simulink model "SF015A_WhlImbRejctn"  (R2013b)
settings: Solver=FixedStepDiscrete  SolverMode=SingleTasking  StartTime=0.0  StopTime=1  FixedStep=0.002  RelTol=1e-3
values from neighbouring files (symbols this model uses):
  ACTIVBANDMAX_ULS_U32 = DataDict.Constant    [SF015A_WhlImbRejctn_DataDict.m]
  ADAPVFILMAX_ULS_F32 = DataDict.Constant    [SF015A_WhlImbRejctn_DataDict.m]
  ARCHGLBPRM_180OVERPI_ULS_F32 = DataDict.Constant    [SF015A_WhlImbRejctn_DataDict.m]
  ARCHGLBPRM_2MILLISEC_SEC_F32 = DataDict.Constant    [SF015A_WhlImbRejctn_DataDict.m]
  ARCHGLBPRM_2PI_ULS_F32 = DataDict.Constant    [SF015A_WhlImbRejctn_DataDict.m]
  ARCHGLBPRM_FLOATZEROTHD_ULS_F32 = DataDict.Constant    [SF015A_WhlImbRejctn_DataDict.m]
  ARCHGLBPRM_PI_ULS_F32 = DataDict.Constant    [SF015A_WhlImbRejctn_DataDict.m]
  ARCHGLBPRM_PIOVER180_ULS_F32 = DataDict.Constant    [SF015A_WhlImbRejctn_DataDict.m]
  ARCHGLBPRM_PIOVER2_ULS_F32 = DataDict.Constant    [SF015A_WhlImbRejctn_DataDict.m]
  CALMINSPERCOUNT_ULS_F32 = DataDict.Constant    [SF015A_WhlImbRejctn_DataDict.m]
  DURATIONDISABLE_CNT_U16 = DataDict.Constant    [SF015A_WhlImbRejctn_DataDict.m]
  FILTWHLSPDMAX_MOTRADPERSEC_F32 = DataDict.Constant    [SF015A_WhlImbRejctn_DataDict.m]
  MICROSECTOMILLISEC_ULS_F32 = DataDict.Constant    [SF015A_WhlImbRejctn_DataDict.m]
  MINSTOMILLISEC_ULS_F32 = DataDict.Constant    [SF015A_WhlImbRejctn_DataDict.m]
  NINETY_ULS_F32 = DataDict.Constant    [SF015A_WhlImbRejctn_DataDict.m]
  NODEBSTEP_CNT_U16 = DataDict.Constant    [SF015A_WhlImbRejctn_DataDict.m]
  NROFDLY_CNT_U08 = DataDict.Constant    [SF015A_WhlImbRejctn_DataDict.m]
  ONEHALF_ULS_F32 = DataDict.Constant    [SF015A_WhlImbRejctn_DataDict.m]
  ONEHUNDRED_ULS_F32 = DataDict.Constant    [SF015A_WhlImbRejctn_DataDict.m]
  ONEOVRTHREE_ULS_F32 = DataDict.Constant    [SF015A_WhlImbRejctn_DataDict.m]
  ONEOVRTWENTY_ULS_F32 = DataDict.Constant    [SF015A_WhlImbRejctn_DataDict.m]
  ONETHOUSAND_ULS_F32 = DataDict.Constant    [SF015A_WhlImbRejctn_DataDict.m]
  PEAKMAX_ULS_F32 = DataDict.Constant    [SF015A_WhlImbRejctn_DataDict.m]
  PEAKMIN_ULS_F32 = DataDict.Constant    [SF015A_WhlImbRejctn_DataDict.m]
  PHAADJMAX_ULS_F32 = DataDict.Constant    [SF015A_WhlImbRejctn_DataDict.m]
  PITIMESSAMPLETIME_ULS_F32 = DataDict.Constant    [SF015A_WhlImbRejctn_DataDict.m]
  STOREDMINSPERCOUNT_ULS_F32 = DataDict.Constant    [SF015A_WhlImbRejctn_DataDict.m]
  TWO_ULS_F32 = DataDict.Constant    [SF015A_WhlImbRejctn_DataDict.m]
  TWOOVRTHREE_ULS_F32 = DataDict.Constant    [SF015A_WhlImbRejctn_DataDict.m]
  WhlImbRejctnAdpvFac = DataDict.Calibration    [SF015A_WhlImbRejctn_DataDict.m]
  WhlImbRejctnAutScaEna = DataDict.Calibration    [SF015A_WhlImbRejctn_DataDict.m]
  WhlImbRejctnAutScaTar = DataDict.Calibration    [SF015A_WhlImbRejctn_DataDict.m]
  WhlImbRejctnCurrMgnSlewPerLoop = DataDict.Calibration    [SF015A_WhlImbRejctn_DataDict.m]
  WhlImbRejctnDcTrendFltRcvryDly = DataDict.Calibration    [SF015A_WhlImbRejctn_DataDict.m]
  WhlImbRejctnDcTrendFltRcvryNegStep = DataDict.Calibration    [SF015A_WhlImbRejctn_DataDict.m]
  WhlImbRejctnDcTrendFltRcvryPosStep = DataDict.Calibration    [SF015A_WhlImbRejctn_DataDict.m]
  WhlImbRejctnDcTrendFltRcvryThd = DataDict.Calibration    [SF015A_WhlImbRejctn_DataDict.m]
  WhlImbRejctnDcTrendTh2Tq = DataDict.Calibration    [SF015A_WhlImbRejctn_DataDict.m]
  WhlImbRejctnDcTrendThTq = DataDict.Calibration    [SF015A_WhlImbRejctn_DataDict.m]
  WhlImbRejctnDcTrendTi2Sec = DataDict.Calibration    [SF015A_WhlImbRejctn_DataDict.m]
  WhlImbRejctnDcTrendTiSec = DataDict.Calibration    [SF015A_WhlImbRejctn_DataDict.m]
  WhlImbRejctnEnaSlewPerLoop = DataDict.Calibration    [SF015A_WhlImbRejctn_DataDict.m]
  WhlImbRejctnFctEna = DataDict.Calibration    [SF015A_WhlImbRejctn_DataDict.m]
  WhlImbRejctnFrqDiagcAmpThd = DataDict.Calibration    [SF015A_WhlImbRejctn_DataDict.m]
  WhlImbRejctnFrqDiagcEna = DataDict.Calibration    [SF015A_WhlImbRejctn_DataDict.m]
  WhlImbRejctnFrqDiagcFltRcvryDly = DataDict.Calibration    [SF015A_WhlImbRejctn_DataDict.m]
  WhlImbRejctnFrqDiagcFltRcvryNegStep = DataDict.Calibration    [SF015A_WhlImbRejctn_DataDict.m]
  WhlImbRejctnFrqDiagcFltRcvryPosStep = DataDict.Calibration    [SF015A_WhlImbRejctn_DataDict.m]
  WhlImbRejctnFrqDiagcFltRcvryThd = DataDict.Calibration    [SF015A_WhlImbRejctn_DataDict.m]
  WhlImbRejctnFrqDiagcThd = DataDict.Calibration    [SF015A_WhlImbRejctn_DataDict.m]
  WhlImbRejctnFrqDiagcTout = DataDict.Calibration    [SF015A_WhlImbRejctn_DataDict.m]
  WhlImbRejctnFrqDiagcUgrPoleMgn = DataDict.Calibration    [SF015A_WhlImbRejctn_DataDict.m]
  WhlImbRejctnFrqScaTblX = DataDict.Calibration    [SF015A_WhlImbRejctn_DataDict.m]
  WhlImbRejctnMaxDurn = DataDict.Calibration    [SF015A_WhlImbRejctn_DataDict.m]
  WhlImbRejctnMaxMgn = DataDict.Calibration    [SF015A_WhlImbRejctn_DataDict.m]
  WhlImbRejctnMaxMgnFltNegStep = DataDict.Calibration    [SF015A_WhlImbRejctn_DataDict.m]
  WhlImbRejctnMaxMgnFltPosStep = DataDict.Calibration    [SF015A_WhlImbRejctn_DataDict.m]
  WhlImbRejctnMaxMgnFltRcvryDly = DataDict.Calibration    [SF015A_WhlImbRejctn_DataDict.m]
  WhlImbRejctnMaxMgnFltRcvryNegStep = DataDict.Calibration    [SF015A_WhlImbRejctn_DataDict.m]
  WhlImbRejctnMaxMgnFltRcvryPosStep = DataDict.Calibration    [SF015A_WhlImbRejctn_DataDict.m]
  WhlImbRejctnMaxMgnFltRcvryThd = DataDict.Calibration    [SF015A_WhlImbRejctn_DataDict.m]
  WhlImbRejctnMaxMgnFltThd = DataDict.Calibration    [SF015A_WhlImbRejctn_DataDict.m]
  WhlImbRejctnMgnEstimnDeltaSca = DataDict.Calibration    [SF015A_WhlImbRejctn_DataDict.m]
  WhlImbRejctnMgnEstimnDiThd = DataDict.Calibration    [SF015A_WhlImbRejctn_DataDict.m]
  WhlImbRejctnMgnEstimnEnaThd = DataDict.Calibration    [SF015A_WhlImbRejctn_DataDict.m]
  WhlImbRejctnMgnEstimnFrq = DataDict.Calibration    [SF015A_WhlImbRejctn_DataDict.m]
  WhlImbRejctnMgnEstimnFrqDelta = DataDict.Calibration    [SF015A_WhlImbRejctn_DataDict.m]
  WhlImbRejctnMgnEstimnLeak = DataDict.Calibration    [SF015A_WhlImbRejctn_DataDict.m]
  WhlImbRejctnRampDwnTi = DataDict.Calibration    [SF015A_WhlImbRejctn_DataDict.m]
  WhlImbRejctnScaCncl = DataDict.Calibration    [SF015A_WhlImbRejctn_DataDict.m]
  WhlImbRejctnUgrPoleMgn = DataDict.Calibration    [SF015A_WhlImbRejctn_DataDict.m]
  WhlImbRejctnVehSpdEna = DataDict.Calibration    [SF015A_WhlImbRejctn_DataDict.m]
  WhlImbRejctnWhlSpdCorrlnFltRcvryDly = DataDict.Calibration    [SF015A_WhlImbRejctn_DataDict.m]
  WhlImbRejctnWhlSpdCorrlnFltRcvryNegStep = DataDict.Calibration    [SF015A_WhlImbRejctn_DataDict.m]
  WhlImbRejctnWhlSpdCorrlnFltRcvryPosStep = DataDict.Calibration    [SF015A_WhlImbRejctn_DataDict.m]
  WhlImbRejctnWhlSpdCorrlnFltRcvryThd = DataDict.Calibration    [SF015A_WhlImbRejctn_DataDict.m]
  WhlImbRejctnWhlSpdCorrlnThd = DataDict.Calibration    [SF015A_WhlImbRejctn_DataDict.m]
  WhlImbRejctnWhlSpdCorrlnTi = DataDict.Calibration    [SF015A_WhlImbRejctn_DataDict.m]
  WIRCMDMAX_MOTNWTMTR_F32 = DataDict.Constant    [SF015A_WhlImbRejctn_DataDict.m]
  ZERO_ULS_F32 = DataDict.Constant    [SF015A_WhlImbRejctn_DataDict.m]
undefined symbols (not defined in the file or in its folder): Cntr, NtcNr1, NvmGetErrSts1, SigQlfr1, Sts, SysSt1
libraries: simulink x32, FixdToFloat x32, Fil x20, NxtrLim x15, NxtrNvM x12, NxtrAbslt x8, NxtrMath x7, NxtrMax x6, NxtrMin x4, FloatToFixd x2, LnrIntrpn x2, NxtrSign x1
(part 1 of 12)
settings Model: Creator=VZBTJX  LastModifiedBy=VZBTJX
settings SolverCC: AutoInsertRateTranBlk=on  InsertRTBMode=Always
settings DataIOCC: LimitDataPoints=off  SaveFormat=Structure  ReturnWorkspaceOutputs=on
settings OptimizationCC: BlockReduction=off  InlineParams=on  ZeroExternalMemoryAtStartup=off  ZeroInternalMemoryAtStartup=off  OptimizeModelRefInitCode=on  LifeSpan=1
settings DebuggingCC: SignalInfNanChecking=error  SignalRangeChecking=warning  UnderspecifiedInitializationDetection=Simplified  SolverPrmCheckMsg=error  InheritedTsInSrcMsg=error  DiscreteInheritContinuousMsg=error  SingleTaskRateTransMsg=error  TasksWithSamePriorityMsg=error  SigSpecEnsureSampleTimeMsg=error  CheckMatrixSingularityMsg=error  ParameterUnderflowMsg=error  ParameterPrecisionLossMsg=error  ParameterTunabilityLossMsg=error  FixptConstUnderflowMsg=warning  FixptConstOverflowMsg=warning  VectorMatrixConversionMsg=error  SignalLabelMismatchMsg=error  UnconnectedInputMsg=error  UnconnectedOutputMsg=error  UnconnectedLineMsg=error  SFcnCompatibilityMsg=error  UniqueDataStoreMsg=warning  BusObjectLabelMismatch=error  RootOutportRequireBusObject=error  AssertControl=DisableAll  ModelReferenceIOMsg=error  ModelReferenceVersionMismatchMessage=warning  ModelReferenceIOMismatchMessage=error  ModelReferenceCSMismatchMessage=warning  ModelReferenceDataLoggingMessage=error  StateNameClashWarn=warning  StrictBusMsg=ErrorOnBusTreatedAsVector  NonBusSignalsTreatedAsBus=error  SFUnexpectedBacktrackingDiag=error  SFInvalidInputDataAccessInChartInitDiag=error  SFNoUnconditionalDefaultTransitionDiag=error  SFTransitionOutsideNaturalParentDiag=error  SFUnconditionalTransitionShadowingDiag=error  SFUndirectedBroadcastEventsDiag=error
settings ModelReferenceCC: ModelReferenceNumInstancesAllowed=Single
settings RTWCC: SystemTargetFile=autosar.tlc  GenCodeOnly=on  TemplateMakefile=ert_default_tmf  Description=AUTOSAR  GenerateReport=on  ProcessScript=autosar_make_rtw_hook  LaunchReport=on
settings CodeAppCC: GenerateComments=off  IgnoreCustomStorageClasses=off  CustomSymbolStrType=$N$R$M  CustomSymbolStrBlkIO=$N$M  SimulinkBlockComments=off
settings STFCustomTargetCC: ParMdlRefBuildCompliant=on  CompOptLevelCompliant=on  IncludeMdlTerminateFcn=off  CombineOutputUpdateFcns=on  SuppressErrorStatus=on  ERTFirstTimeCompliant=on  ERTCustomFileBanners=on  SupportNonFinite=off  SupportComplex=off  SupportContinuousTime=off  SupportNonInlinedSFcns=off  MATLABClassNameForMDSCustomization=Simulink.SoftwareTarget.ERTCustomization  AutosarCompliant=on  GRTInterface=off  SystemTargetFile=autosar.tlc
settings ERTTargetCC: CodeReplacementLibrary=ANSI_C  ConcurrentExecutionCompliant=off  IncludeMdlTerminateFcn=off  SuppressErrorStatus=on  SupportNonFinite=off  SupportComplex=off  ModelStepFunctionPrototypeControlCompliant=off  CPPClassGenCompliant=off  AutosarCompliant=on  InlinedParameterPlacement=NonHierarchical  ERTCustomFileTemplate=example_file_process.tlc  EnableUserReplacementTypes=on

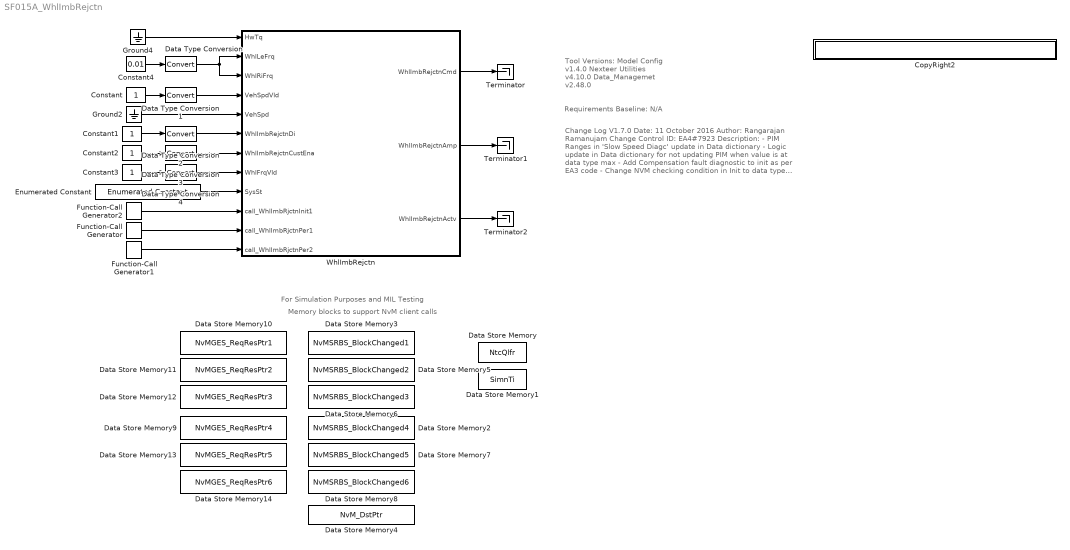
== system SF015A_WhlImbRejctn ==
  note: Requirements Baseline: N/A
  note: Tool Versions:
      |
      | Model Config v1.4.0
      | Nexteer Utilities v4.10.0
      | Data_Managemet v2.48.0
  note: Change Log
      |
      | V1.7.0
      | Date: 11 October 2016
      | Author: Rangarajan Ramanujam
      | Change Control ID: EA4#7923
      | Description:
      | - PIM Ranges in 'Slow Speed Diagc' update in Data dictionary
      | - Logic update in Data dictionary for not updating PIM when value is at
      | data type max
      | - Add Compensation fault diagnostic to init as per EA3 code
      | - Change NVM checking condition in Init to data type max of u32 instead of
      | u16
      | -The Lowpass filter variable for computing CurrMagLe and CurrMagRi
      | were same and this was resolved with separate Low pass filter state
      | variables for Le and Ri.
      | - Logic for Enabling and disabling WIR updated/changed as per Ea3 code
      |
      | V1.6.0
      | - Minimum Value of LpFil variables checked and changed to prevent
      |  divide by zero issues
      | - Latest tools used to fix LpFil error and prevent LpFilGain being
      | set to zero
      | - Display variable write blocks missing were updated :
      | dWhlImbRejctnLMSqdOutLe and dWhlImbRejctnLMSqdOutRi
      | - Pim Data store memory blocks Diagnostics set to 'none'
      | - Width block used to select first and last elements of an array
      | instead of using 'Arrayname(1)' or 'Arrayname(end)'
      |
      | V1.5.0
      | - 'OR' block replaced with 'Bitwise OR' in the subsystem 'WIR
      | Diagnostics/Set NTC Block'.
      | - Updated the datatype of NTC failure bits to 'uint8' in the 'WIR
      | Diagnostics/Set NTC Block'.
      | - Logic for setting of NTC bit based on WheelFrequencyValid
      | signal has been removed from the subsystem 'WIR Diagnostics'.
      | - Properties of few simulink blocks have been changed to make
      | the model simulatable.
      | - The definition of PIMs of type'Bus:PassFailCntrDiagcRec1' has
      | been updated in the data dictionary.
      |
      |
      | V1.4.0
      | Date: 01 August 2016
      | Author: Rangarajan Ramanujam
      | Change Control: 6681
      | Description:
      | - Rearranging design logic in Wheel speed Correlation check
      |  to remove redundant checks and  match code with model
      |
      | v1.3.0
      | Date: 6 June 2016
      | Author: Sneha Singh
      | Change Control ID: EA4# 5952
      | - NOT block added to the signal WhlImbRejctnDi
      | - Elapsed timer comparison modified from '<=' to '>='.
      | - Changed units of few cals from 'Milliseconds' to 'Mins'.
      | - Logic for conversion of minutes to milliseconds added.
      | - Added a new constant for minutes to milliseconds conversion.
      |
      | V1.2.0
      | Date: 23 Mar 2016
      | Author :Rangarajan Ramanujam
      | Change control :
      | Description:
      | - NVM checks added
      | - Typos fixed in cal names
      | - Design changes in Phase adjust
      | - Initial values updated according to review
      |
      | V1.1.0
      | -Changes corresponding to software review
      |
      | V1.0.0
      | - Initial Release
      | - Based on EA3 Word doc
      | - Level 3 Model
  note: For Simulation Purposes and MIL Testing
  note: Memory blocks to support NvM client calls
  Constant{,1..3} (4 alike) : Constant
  Constant4 : Constant  Value=0.01
  CopyRight2 : Subsystem  Description=|  mask(Copyright Information){none=on}
      | Copyright info block.                                               
      |                                                                     
      | Place copyright information at the top of every subsystem in design.
      mask prompts: none "No parameters"
      mask help: Place copyright information at the top of every subsystem in design.
      mask Display:
      | NxtrConf = 'Nexteer Confidential';
      | 
      | sys = bdroot; %handle for the current model ("system")
      | first = get_param(sys,'Created');
      | first = first(end-3:end);  %year is last four digits
      | 
      | last = get_param(sys,'LastModifiedDate');
      | if isempty(last)
      |     last = datestr(now,'yyyy');
      | else
      |     last = last(end-3:end);
      | end
      | 
      | if strcmp(first,last)
      |     fprintf('%s -- Copyright %s Nexteer',NxtrConf,first)
      | else
      |     fprintf('%s -- %s%s- %s Nexteer',NxtrConf,char(169),first,last)
      | end
  Data Store Memory : DataStoreMemory  DataStoreName=NtcQlfr
  Data Store Memory1 : DataStoreMemory  DataStoreName=SimnTi
  Data Store Memory10 : DataStoreMemory  DataStoreName=NvMGES_ReqResPtr1
  Data Store Memory11 : DataStoreMemory  DataStoreName=NvMGES_ReqResPtr2
  Data Store Memory12 : DataStoreMemory  DataStoreName=NvMGES_ReqResPtr3
  Data Store Memory13 : DataStoreMemory  DataStoreName=NvMGES_ReqResPtr5
  Data Store Memory14 : DataStoreMemory  DataStoreName=NvMGES_ReqResPtr6
  Data Store Memory2 : DataStoreMemory  DataStoreName=NvMSRBS_BlockChanged4
  Data Store Memory3 : DataStoreMemory  DataStoreName=NvMSRBS_BlockChanged1
  Data Store Memory4 : DataStoreMemory  DataStoreName=NvM_DstPtr
  Data Store Memory5 : DataStoreMemory  DataStoreName=NvMSRBS_BlockChanged2
  Data Store Memory6 : DataStoreMemory  DataStoreName=NvMSRBS_BlockChanged3
  Data Store Memory7 : DataStoreMemory  DataStoreName=NvMSRBS_BlockChanged5
  Data Store Memory8 : DataStoreMemory  DataStoreName=NvMSRBS_BlockChanged6
  Data Store Memory9 : DataStoreMemory  DataStoreName=NvMGES_ReqResPtr4
  Data Type Conversion{,1..4} (5 alike) : DataTypeConversion
  Enumerated Constant : simulink/Sources/Enumerated Constant  OutDataTypeStr=Enum: SysSt1  Value=SysSt1.SYSST_WRMININ  SampleTime=inf
  Function-Call Generator : simulink/Ports & Subsystems/Function-Call Generator  sample_time=0.002  numberOfIterations=1
  Function-Call Generator1 : simulink/Ports & Subsystems/Function-Call Generator  sample_time=0.01  numberOfIterations=1
  Function-Call Generator2 : simulink/Ports & Subsystems/Function-Call Generator  sample_time=0  numberOfIterations=1
  Ground2 : Ground
  Ground4 : Ground
  Terminator : Terminator
  Terminator1 : Terminator
  Terminator2 : Terminator
  WhlImbRejctn : Subsystem
  wires:
  WhlImbRejctn/1(WhlImbRejctnCmd) -> Terminator/1
  WhlImbRejctn/2(WhlImbRejctnAmp) -> Terminator1/1
  Ground4/1 -> WhlImbRejctn/1(HwTq)
  Constant4/1 -> Data Type Conversion/1
  Constant/1 -> Data Type Conversion1/1
  Ground2/1 -> WhlImbRejctn/5(VehSpd)
  Constant1/1 -> Data Type Conversion2/1
  Constant2/1 -> Data Type Conversion3/1
  Constant3/1 -> Data Type Conversion4/1
  Function-Call Generator/1 -> WhlImbRejctn/11(call_WhlImbRjctnPer1)
  Function-Call Generator2/1 -> WhlImbRejctn/10(call_WhlImbRjctnInit1)
  Enumerated Constant/1 -> WhlImbRejctn/9(SysSt)
  Function-Call Generator1/1 -> WhlImbRejctn/12(call_WhlImbRjctnPer2)
  WhlImbRejctn/3(WhlImbRejctnActv) -> Terminator2/1
  Data Type Conversion/1 -> WhlImbRejctn/2(WhlLeFrq), WhlImbRejctn/3(WhlRiFrq)
  Data Type Conversion1/1 -> WhlImbRejctn/4(VehSpdVld)
  Data Type Conversion2/1 -> WhlImbRejctn/6(WhlImbRejctnDi)
  Data Type Conversion3/1 -> WhlImbRejctn/7(WhlImbRejctnCustEna)
  Data Type Conversion4/1 -> WhlImbRejctn/8(WhlFrqVld)

== system SF015A_WhlImbRejctn/CopyRight2 ==

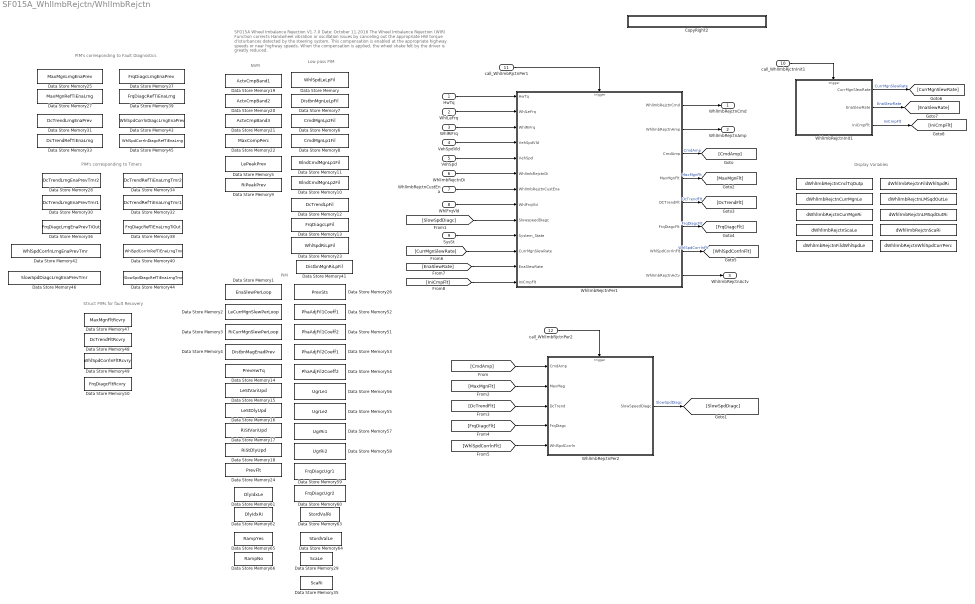
== system SF015A_WhlImbRejctn/WhlImbRejctn ==
  note: Struct PIMs for fault Recovery
  note: PIM's corresponding to Timers
  note: PIM's corresponding to Fault Diagnostics
  note: NVM
  note: PIM
  note: Display Variables
  note: Low pass PIM
  note: SF015A Wheel Imbalance Rejection
      | V1.7.0 																													    Date: October 11,2016
      |
      | The Wheel Imbalance Rejection (WIR) Function corrects Handwheel vibration or oscillation issues by canceling out the appropriate HW torque
      | d'isturbances detected by the steering system. This compensation is enabled at the appropriate highway speeds or near highway speeds. When the
      | compensation is applied, the wheel shake felt by the driver is greatly reduced.
  HwTq : Inport
  WhlLeFrq : Inport  Port=2
  WhlRiFrq : Inport  Port=3
  VehSpdVld : Inport  Port=4
  VehSpd : Inport  Port=5
  WhlImbRejctnDi : Inport  Port=6
  WhlImbRejctnCustEna : Inport  Port=7
  WhlFrqVld : Inport  Port=8
  SysSt : Inport  Port=9
  call_WhlImbRjctnInit1 : Inport  Port=10
  call_WhlImbRjctnPer1 : Inport  Port=11
  call_WhlImbRjctnPer2 : Inport  Port=12
  " " : DataStoreMemory  DataStoreName=dWhlImbRejctnCnclTqOutp  StateMustResolveToSignalObject=on
  " " : DataStoreMemory  DataStoreName=dWhlImbRejctnCurrMgnLe  StateMustResolveToSignalObject=on
  " " : DataStoreMemory  DataStoreName=dWhlImbRejctnCurrMgnRi  StateMustResolveToSignalObject=on
  " " : DataStoreMemory  DataStoreName=dWhlImbRejctnFildWhlSpdLe  StateMustResolveToSignalObject=on
  " " : DataStoreMemory  DataStoreName=dWhlImbRejctnFildWhlSpdRi  StateMustResolveToSignalObject=on
  " " : DataStoreMemory  DataStoreName=dWhlImbRejctnLMSqdOutLe  StateMustResolveToSignalObject=on
  " " : DataStoreMemory  DataStoreName=dWhlImbRejctnLMSqdOutRi  StateMustResolveToSignalObject=on
  " " : DataStoreMemory  DataStoreName=dWhlImbRejctnScaLe  StateMustResolveToSignalObject=on
  " " : DataStoreMemory  DataStoreName=dWhlImbRejctnScaRi  StateMustResolveToSignalObject=on
  " " : DataStoreMemory  DataStoreName=dWhlImbRejctnWhlSpdCorrPerc  StateMustResolveToSignalObject=on
  CopyRight2 : Subsystem  Description=|  mask(Copyright Information){none=on}
      | Copyright info block.                                               
      |                                                                     
      | Place copyright information at the top of every subsystem in design.
      mask prompts: none "No parameters"
      mask help: Place copyright information at the top of every subsystem in design.
      mask Display:
      | NxtrConf = 'Nexteer Confidential';
      | 
      | sys = bdroot; %handle for the current model ("system")
      | first = get_param(sys,'Created');
      | first = first(end-3:end);  %year is last four digits
      | 
      | last = get_param(sys,'LastModifiedDate');
      | if isempty(last)
      |     last = datestr(now,'yyyy');
      | else
      |     last = last(end-3:end);
      | end
      | 
      | if strcmp(first,last)
      |     fprintf('%s -- Copyright %s Nexteer',NxtrConf,first)
      | else
      |     fprintf('%s -- %s%s- %s Nexteer',NxtrConf,char(169),first,last)
      | end
  Data Store Memory : DataStoreMemory  DataStoreName=WhlSpdLeLpFil  InitialValue=[]  OutDataTypeStr=Bus: FilLpRec1  StateMustResolveToSignalObject=on
  Data Store Memory1 : DataStoreMemory  DataStoreName=EnaSlewPerLoop  InitialValue=[]  StateMustResolveToSignalObject=on
  Data Store Memory10 : DataStoreMemory  DataStoreName=BlndCmdMgnLp2Fil  InitialValue=[]  OutDataTypeStr=Bus: FilLpRec1  StateMustResolveToSignalObject=on
  Data Store Memory11 : DataStoreMemory  DataStoreName=BlndCmdMgnLp1Fil  InitialValue=[]  OutDataTypeStr=Bus: FilLpRec1  StateMustResolveToSignalObject=on
  Data Store Memory12 : DataStoreMemory  DataStoreName=DcTrendLpFil  InitialValue=[]  OutDataTypeStr=Bus: FilLpRec1  StateMustResolveToSignalObject=on
  Data Store Memory13 : DataStoreMemory  DataStoreName=FrqDiagcLpFil  InitialValue=[]  OutDataTypeStr=Bus: FilLpRec1  StateMustResolveToSignalObject=on
  Data Store Memory14 : DataStoreMemory  DataStoreName=PrevHwTq  InitialValue=[]  StateMustResolveToSignalObject=on
  Data Store Memory15 : DataStoreMemory  DataStoreName=LeStVariUpd  InitialValue=[]  StateMustResolveToSignalObject=on
  Data Store Memory16 : DataStoreMemory  DataStoreName=LeStDlyUpd  InitialValue=[]  StateMustResolveToSignalObject=on
  Data Store Memory17 : DataStoreMemory  DataStoreName=RiStVariUpd  InitialValue=[]  StateMustResolveToSignalObject=on
  Data Store Memory18 : DataStoreMemory  DataStoreName=RiStDlyUpd  InitialValue=[]  StateMustResolveToSignalObject=on
  Data Store Memory19 : DataStoreMemory  DataStoreName=ActvCmpBand1  InitialValue=[]  StateMustResolveToSignalObject=on
  Data Store Memory2 : DataStoreMemory  DataStoreName=LeCurrMgnSlewPerLoop  InitialValue=[]  StateMustResolveToSignalObject=on
  Data Store Memory20 : DataStoreMemory  DataStoreName=ActvCmpBand2  InitialValue=[]  StateMustResolveToSignalObject=on
  Data Store Memory21 : DataStoreMemory  DataStoreName=ActvCmpBand3  InitialValue=[]  StateMustResolveToSignalObject=on
  Data Store Memory22 : DataStoreMemory  DataStoreName=MaxCompPerc  InitialValue=[]  StateMustResolveToSignalObject=on
  Data Store Memory23 : DataStoreMemory  DataStoreName=WhlSpdRiLpFil  InitialValue=[]  OutDataTypeStr=Bus: FilLpRec1  StateMustResolveToSignalObject=on
  Data Store Memory24 : DataStoreMemory  DataStoreName=PrevFlt  InitialValue=[]  StateMustResolveToSignalObject=on
  Data Store Memory25 : DataStoreMemory  DataStoreName=MaxMgnLrngEnaPrev  InitialValue=[]  StateMustResolveToSignalObject=on
  Data Store Memory26 : DataStoreMemory  DataStoreName=PrevSts  InitialValue=[]  StateMustResolveToSignalObject=on
  Data Store Memory27 : DataStoreMemory  DataStoreName=MaxMgnRefTiEnaLrng  InitialValue=[]  StateMustResolveToSignalObject=on
  Data Store Memory28 : DataStoreMemory  DataStoreName=DcTrendLrngEnaPrevTmr2  InitialValue=[]  StateMustResolveToSignalObject=on
  Data Store Memory29 : DataStoreMemory  DataStoreName=ScaLe  StateMustResolveToSignalObject=on
  Data Store Memory3 : DataStoreMemory  DataStoreName=RiCurrMgnSlewPerLoop  InitialValue=[]  StateMustResolveToSignalObject=on
  Data Store Memory30 : DataStoreMemory  DataStoreName=DcTrendLrngEnaPrevTmr1  InitialValue=[]  StateMustResolveToSignalObject=on
  Data Store Memory31 : DataStoreMemory  DataStoreName=DcTrendLrngEnaPrev  InitialValue=[]  StateMustResolveToSignalObject=on
  Data Store Memory32 : DataStoreMemory  DataStoreName=DcTrendRefTiEnaLrngTmr1  InitialValue=[]  StateMustResolveToSignalObject=on
  Data Store Memory33 : DataStoreMemory  DataStoreName=DcTrendRefTiEnaLrng  InitialValue=[]  StateMustResolveToSignalObject=on
  Data Store Memory34 : DataStoreMemory  DataStoreName=DcTrendRefTiEnaLrngTmr2  InitialValue=[]  StateMustResolveToSignalObject=on
  Data Store Memory35 : DataStoreMemory  DataStoreName=ScaRi  StateMustResolveToSignalObject=on
  Data Store Memory36 : DataStoreMemory  DataStoreName=FrqDiagcLrngEnaPrevTiOut  InitialValue=[]  StateMustResolveToSignalObject=on
  Data Store Memory37 : DataStoreMemory  DataStoreName=FrqDiagcLrngEnaPrev  InitialValue=[]  StateMustResolveToSignalObject=on
  Data Store Memory38 : DataStoreMemory  DataStoreName=FrqDiagcRefTiEnaLrngTiOut  InitialValue=[]  StateMustResolveToSignalObject=on
  Data Store Memory39 : DataStoreMemory  DataStoreName=FrqDiagcRefTiEnaLrng  InitialValue=[]  StateMustResolveToSignalObject=on
  Data Store Memory4 : DataStoreMemory  DataStoreName=DistbnMagEnadPrev  InitialValue=[]  StateMustResolveToSignalObject=on
  Data Store Memory40 : DataStoreMemory  DataStoreName=WhlSpdCorrlnRefTiEnaLrngTmr  InitialValue=[]  StateMustResolveToSignalObject=on
  Data Store Memory41 : DataStoreMemory  DataStoreName=DistbnMgnRiLpFil  InitialValue=[]  OutDataTypeStr=Bus: FilLpRec1  StateMustResolveToSignalObject=on
  Data Store Memory42 : DataStoreMemory  DataStoreName=WhlSpdCorrlnLrngEnaPrevTmr  InitialValue=[]  StateMustResolveToSignalObject=on
  Data Store Memory43 : DataStoreMemory  DataStoreName=WhlSpdCorrlnDiagcLrngEnaPrev  InitialValue=[]  StateMustResolveToSignalObject=on
  Data Store Memory44 : DataStoreMemory  DataStoreName=SlowSpdDiagcRefTiEnaLrngTmr  InitialValue=[]  StateMustResolveToSignalObject=on
  Data Store Memory45 : DataStoreMemory  DataStoreName=WhlSpdCorrlnDiagcRefTiEnaLrng  InitialValue=[]  StateMustResolveToSignalObject=on
  Data Store Memory46 : DataStoreMemory  DataStoreName=SlowSpdDiagcLrngEnaPrevTmr  InitialValue=[]  StateMustResolveToSignalObject=on
  Data Store Memory47 : DataStoreMemory  DataStoreName=MaxMgnFltRcvry  InitialValue=[]  OutDataTypeStr=Bus:PassFailCntrDiagcRec1  StateMustResolveToSignalObject=on
  Data Store Memory48 : DataStoreMemory  DataStoreName=DcTrendFltRcvry  InitialValue=[]  OutDataTypeStr=Bus: PassFailCntrDiagcRec1  StateMustResolveToSignalObject=on
  Data Store Memory49 : DataStoreMemory  DataStoreName=WhlSpdCorrlnFltRcvry  InitialValue=[]  OutDataTypeStr=Bus: PassFailCntrDiagcRec1  StateMustResolveToSignalObject=on
  Data Store Memory5 : DataStoreMemory  DataStoreName=LePeakPrev  InitialValue=[]  StateMustResolveToSignalObject=on
  Data Store Memory50 : DataStoreMemory  DataStoreName=FrqDiagcFltRcvry  InitialValue=[]  OutDataTypeStr=Bus: PassFailCntrDiagcRec1  StateMustResolveToSignalObject=on
  Data Store Memory51 : DataStoreMemory  DataStoreName=PhaAdjFil1Coeff2  InitialValue=[]  StateMustResolveToSignalObject=on
  Data Store Memory52 : DataStoreMemory  DataStoreName=PhaAdjFil1Coeff1  InitialValue=[]  StateMustResolveToSignalObject=on
  Data Store Memory53 : DataStoreMemory  DataStoreName=PhaAdjFil2Coeff1  InitialValue=[]  StateMustResolveToSignalObject=on
  Data Store Memory54 : DataStoreMemory  DataStoreName=PhaAdjFil2Coeff2  InitialValue=[]  StateMustResolveToSignalObject=on
  Data Store Memory55 : DataStoreMemory  DataStoreName=UgrLe2  InitialValue=[]  StateMustResolveToSignalObject=on
  Data Store Memory56 : DataStoreMemory  DataStoreName=UgrLe1  InitialValue=[]  StateMustResolveToSignalObject=on
  Data Store Memory57 : DataStoreMemory  DataStoreName=UgrRi1  InitialValue=[]  StateMustResolveToSignalObject=on
  Data Store Memory58 : DataStoreMemory  DataStoreName=UgrRi2  InitialValue=[]  StateMustResolveToSignalObject=on
  Data Store Memory59 : DataStoreMemory  DataStoreName=FrqDiagcUgr1  InitialValue=[]  StateMustResolveToSignalObject=on
  Data Store Memory6 : DataStoreMemory  DataStoreName=CmdMgnLp2Fil  InitialValue=[]  OutDataTypeStr=Bus: FilLpRec1  StateMustResolveToSignalObject=on
  Data Store Memory60 : DataStoreMemory  DataStoreName=FrqDiagcUgr2  InitialValue=[]  StateMustResolveToSignalObject=on
  Data Store Memory61 : DataStoreMemory  DataStoreName=DlyIdxLe  StateMustResolveToSignalObject=on
  Data Store Memory62 : DataStoreMemory  DataStoreName=DlyIdxRi  StateMustResolveToSignalObject=on
  Data Store Memory63 : DataStoreMemory  DataStoreName=StordValRi  InitialValue=[]  StateMustResolveToSignalObject=on
  Data Store Memory64 : DataStoreMemory  DataStoreName=StordValLe  InitialValue=[]  StateMustResolveToSignalObject=on
  Data Store Memory65 : DataStoreMemory  DataStoreName=RampYes  StateMustResolveToSignalObject=on
  Data Store Memory66 : DataStoreMemory  DataStoreName=RampNo  StateMustResolveToSignalObject=on
  Data Store Memory7 : DataStoreMemory  DataStoreName=DistbnMgnLeLpFil  InitialValue=[]  OutDataTypeStr=Bus: FilLpRec1  StateMustResolveToSignalObject=on
  Data Store Memory8 : DataStoreMemory  DataStoreName=CmdMgnLp1Fil  InitialValue=[]  OutDataTypeStr=Bus: FilLpRec1  StateMustResolveToSignalObject=on
  Data Store Memory9 : DataStoreMemory  DataStoreName=RiPeakPrev  InitialValue=[]  StateMustResolveToSignalObject=on
  WhlImbRejctnInit1 : Subsystem
  WhlImbRejctnPer1 : Subsystem
  WhlImbRejctnPer2 : Subsystem  TreatAsAtomicUnit=on
  WhlImbRejctnCmd : Outport
  WhlImbRejctnAmp : Outport  Port=2
  WhlImbRejctnActv : Outport  Port=3
  wires:
  WhlLeFrq/1 -> WhlImbRejctnPer1/2(WhlLeFrq)
  WhlRiFrq/1 -> WhlImbRejctnPer1/3(WhlRiFrq)
  VehSpdVld/1 -> WhlImbRejctnPer1/4(VehSpdVld)
  WhlImbRejctnDi/1 -> WhlImbRejctnPer1/6(WhlImbRejctnDi)
  VehSpd/1 -> WhlImbRejctnPer1/5(VehSpd)
  WhlImbRejctnCustEna/1 -> WhlImbRejctnPer1/7(WhlImbRejctnCustEna)
  HwTq/1 -> WhlImbRejctnPer1/1(HwTq)
  WhlImbRejctnPer1/1(WhlImbRejctnCmd) -> WhlImbRejctnCmd/1
  WhlImbRejctnPer1/2(WhlImbRejctnAmp) -> WhlImbRejctnAmp/1
  call_WhlImbRjctnInit1/1 -> WhlImbRejctnInit1/Trigger
  call_WhlImbRjctnPer1/1 -> WhlImbRejctnPer1/Trigger
  WhlFrqVld/1 -> WhlImbRejctnPer1/8(WhlFrqVld)
  call_WhlImbRjctnPer2/1 -> WhlImbRejctnPer2/Trigger
  WhlImbRejctnPer1/3(CmdAmp) -> [CmdAmp]  "CmdAmp"
  [CmdAmp] -> WhlImbRejctnPer2/1(CmdAmp)
  WhlImbRejctnPer2/1("SlowSpeedDiagc ") -> [SlowSpdDiagc]  "SlowSpdDiagc"
  [SlowSpdDiagc] -> WhlImbRejctnPer1/9(SlowspeedDiagc)
  SysSt/1 -> WhlImbRejctnPer1/10(System_State)
  WhlImbRejctnPer1/7(WhlSpdCorrlnFlt) -> [WhlSpdCorrlnFlt]  "WhlSpdCorrlnFlt"
  WhlImbRejctnPer1/6(FrqDiagcFlt) -> [FrqDiagcFlt]  "FrqDiagcFlt"
  WhlImbRejctnPer1/5(DCTrendFlt) -> [DcTrendFlt]  "DcTrendFlt"
  WhlImbRejctnPer1/4(MaxMgnFlt) -> [MaxMgnFlt]  "MaxMgnFlt"
  [MaxMgnFlt] -> WhlImbRejctnPer2/2(MaxMag)
  [DcTrendFlt] -> WhlImbRejctnPer2/3(DcTrend)
  [FrqDiagcFlt] -> WhlImbRejctnPer2/4(FrqDiagc)
  [WhlSpdCorrlnFlt] -> WhlImbRejctnPer2/5(WhlSpdCorrln)
  WhlImbRejctnPer1/8(WhlImbRejctnActv) -> WhlImbRejctnActv/1
  WhlImbRejctnInit1/1(CurrMgnSlewRate) -> [CurrMgnSlewRate]  "CurrMgnSlewRate"
  [CurrMgnSlewRate] -> WhlImbRejctnPer1/11(CurrMgnSlewRate)
  [EnaSlewRate] -> WhlImbRejctnPer1/12(EnaSlewRate)
  WhlImbRejctnInit1/2(EnaSlewRate) -> [EnaSlewRate]  "EnaSlewRate"
  WhlImbRejctnInit1/3(IniCmpFlt) -> [IniCmpFlt]  "IniCmpFlt"
  [IniCmpFlt] -> WhlImbRejctnPer1/13(IniCmpFlt)

== system SF015A_WhlImbRejctn/WhlImbRejctn/CopyRight2 ==

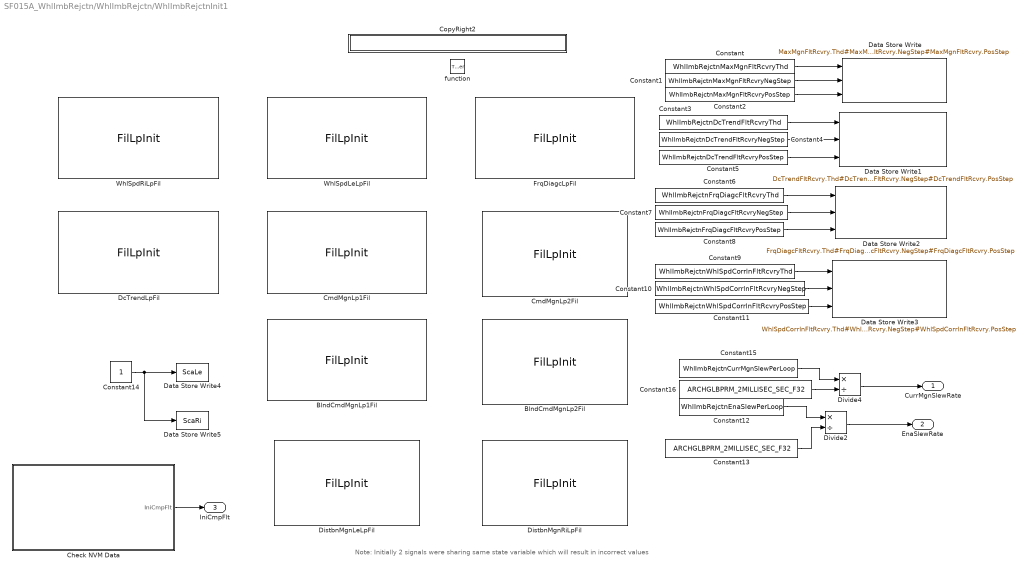
== system SF015A_WhlImbRejctn/WhlImbRejctn/WhlImbRejctnInit1 ==
  note: Note: Initially 2 signals were sharing same state variable which will result in incorrect values
  function : TriggerPort  TriggerType=function-call
  BlndCmdMgnLp1Fil : Fil/FilLpInit  Ic=0  Ts=ARCHGLBPRM_2MILLISEC_SEC_F32  Freq=WhlImbRejctnBlndCmdMgnLp1FilFrq  StVar=BlndCmdMgnLp1Fil
  BlndCmdMgnLp2Fil : Fil/FilLpInit  Ic=0  Ts=ARCHGLBPRM_2MILLISEC_SEC_F32  Freq=WhlImbRejctnBlndCmdMgnLp2FilFrq  StVar=BlndCmdMgnLp2Fil
  Check NVM Data : Subsystem
  CmdMgnLp1Fil : Fil/FilLpInit  Ic=0  Ts=ARCHGLBPRM_2MILLISEC_SEC_F32  Freq=WhlImbRejctnCmdMgnLp1FilFrq  StVar=CmdMgnLp1Fil
  CmdMgnLp2Fil : Fil/FilLpInit  Ic=0  Ts=ARCHGLBPRM_2MILLISEC_SEC_F32  Freq=WhlImbRejctnCmdMgnLp2FilFrq  StVar=CmdMgnLp2Fil
  Constant : Constant  Value=WhlImbRejctnMaxMgnFltRcvryThd
  Constant1 : Constant  Value=WhlImbRejctnMaxMgnFltRcvryNegStep
  Constant10 : Constant  Value=WhlImbRejctnWhlSpdCorrlnFltRcvryNegStep
  Constant11 : Constant  Value=WhlImbRejctnWhlSpdCorrlnFltRcvryPosStep
  Constant12 : Constant  Value=WhlImbRejctnEnaSlewPerLoop
  Constant13 : Constant  Value=ARCHGLBPRM_2MILLISEC_SEC_F32
  Constant14 : Constant  OutDataTypeStr=single
  Constant15 : Constant  Value=WhlImbRejctnCurrMgnSlewPerLoop
  Constant16 : Constant  Value=ARCHGLBPRM_2MILLISEC_SEC_F32
  Constant2 : Constant  Value=WhlImbRejctnMaxMgnFltRcvryPosStep  OutDataTypeStr=single
  Constant3 : Constant  Value=WhlImbRejctnDcTrendFltRcvryThd
  Constant4 : Constant  Value=WhlImbRejctnDcTrendFltRcvryNegStep
  Constant5 : Constant  Value=WhlImbRejctnDcTrendFltRcvryPosStep
  Constant6 : Constant  Value=WhlImbRejctnFrqDiagcFltRcvryThd
  Constant7 : Constant  Value=WhlImbRejctnFrqDiagcFltRcvryNegStep
  Constant8 : Constant  Value=WhlImbRejctnFrqDiagcFltRcvryPosStep
  Constant9 : Constant  Value=WhlImbRejctnWhlSpdCorrlnFltRcvryThd
  CopyRight2 : Subsystem  Description=|  mask(Copyright Information){none=on}
      | Copyright info block.                                               
      |                                                                     
      | Place copyright information at the top of every subsystem in design.
      mask prompts: none "No parameters"
      mask help: Place copyright information at the top of every subsystem in design.
      mask Display:
      | NxtrConf = 'Nexteer Confidential';
      | 
      | sys = bdroot; %handle for the current model ("system")
      | first = get_param(sys,'Created');
      | if(isempty(first))
      |     first = datestr(now,'yyyy');
      | else
      |     first = first(end-3:end);  %year is last four digits
      | end
      | 
      | last = get_param(sys,'LastModifiedDate');
      | if isempty(last)
      |     last = datestr(now,'yyyy');
      | else
      |     last = last(end-3:end);
      | end
      | 
      | if strcmp(first,last)
      |     fprintf('%s -- Copyright %s Nexteer',NxtrConf,first)
      | else
      |     fprintf('%s -- %s%s- %s Nexteer',NxtrConf,char(169),first,last)
      | end
  Data Store Write : DataStoreWrite  DataStoreName=MaxMgnFltRcvry  DataStoreElements=MaxMgnFltRcvry.Thd#MaxMgnFltRcvry.NegStep#MaxMgnFltRcvry.PosStep
  Data Store Write1 : DataStoreWrite  DataStoreName=DcTrendFltRcvry  DataStoreElements=DcTrendFltRcvry.Thd#DcTrendFltRcvry.NegStep#DcTrendFltRcvry.PosStep
  Data Store Write2 : DataStoreWrite  DataStoreName=FrqDiagcFltRcvry  DataStoreElements=FrqDiagcFltRcvry.Thd#FrqDiagcFltRcvry.NegStep#FrqDiagcFltRcvry.PosStep
  Data Store Write3 : DataStoreWrite  DataStoreName=WhlSpdCorrlnFltRcvry  DataStoreElements=WhlSpdCorrlnFltRcvry.Thd#WhlSpdCorrlnFltRcvry.NegStep#WhlSpdCorrlnFltRcvry.PosStep
  Data Store Write4 : DataStoreWrite  DataStoreName=ScaLe
      settings: AttributesFormatString=%<Priority>
  Data Store Write5 : DataStoreWrite  DataStoreName=ScaRi
      settings: AttributesFormatString=%<Priority>
  DcTrendLpFil : Fil/FilLpInit  Ic=0  Ts=ARCHGLBPRM_2MILLISEC_SEC_F32  Freq=WhlImbRejctnDcTrendLpFil  StVar=DcTrendLpFil
  DistbnMgnLeLpFil : Fil/FilLpInit  Ic=0  Ts=ARCHGLBPRM_2MILLISEC_SEC_F32  Freq=WhlImbRejctnDistbnMgnLpFil  StVar=DistbnMgnLeLpFil
  DistbnMgnRiLpFil : Fil/FilLpInit  Ic=0  Ts=ARCHGLBPRM_2MILLISEC_SEC_F32  Freq=WhlImbRejctnDistbnMgnLpFil  StVar=DistbnMgnRiLpFil
  Divide2 : Product  Inputs=*/
  Divide4 : Product  Inputs=*/
  FrqDiagcLpFil : Fil/FilLpInit  Ic=0  Ts=ARCHGLBPRM_2MILLISEC_SEC_F32  Freq=WhlImbRejctnFrqDiagcLpFil  StVar=FrqDiagcLpFil
  WhlSpdLeLpFil : Fil/FilLpInit  Ic=0  Ts=ARCHGLBPRM_2MILLISEC_SEC_F32  Freq=WhlImbRejctnWhlSpdLpFil  StVar=WhlSpdLeLpFil
  WhlSpdRiLpFil : Fil/FilLpInit  Ic=0  Ts=ARCHGLBPRM_2MILLISEC_SEC_F32  Freq=WhlImbRejctnWhlSpdLpFil  StVar=WhlSpdRiLpFil
  CurrMgnSlewRate : Outport
  EnaSlewRate : Outport  Port=2
  IniCmpFlt : Outport  Port=3
  wires:
  Constant15/1 -> Divide4/1
  Constant16/1 -> Divide4/2
  Divide4/1 -> CurrMgnSlewRate/1
  Constant12/1 -> Divide2/1
  Constant13/1 -> Divide2/2
  Divide2/1 -> EnaSlewRate/1
  Constant14/1 -> Data Store Write5/1, Data Store Write4/1
  Constant/1 -> Data Store Write/1
  Constant1/1 -> Data Store Write/2
  Constant2/1 -> Data Store Write/3
  Constant5/1 -> Data Store Write1/3
  Constant4/1 -> Data Store Write1/2
  Constant3/1 -> Data Store Write1/1
  Constant7/1 -> Data Store Write2/2
  Constant8/1 -> Data Store Write2/3
  Constant6/1 -> Data Store Write2/1
  Constant11/1 -> Data Store Write3/3
  Constant10/1 -> Data Store Write3/2
  Constant9/1 -> Data Store Write3/1
  Check NVM Data/1(IniCmpFlt) -> IniCmpFlt/1

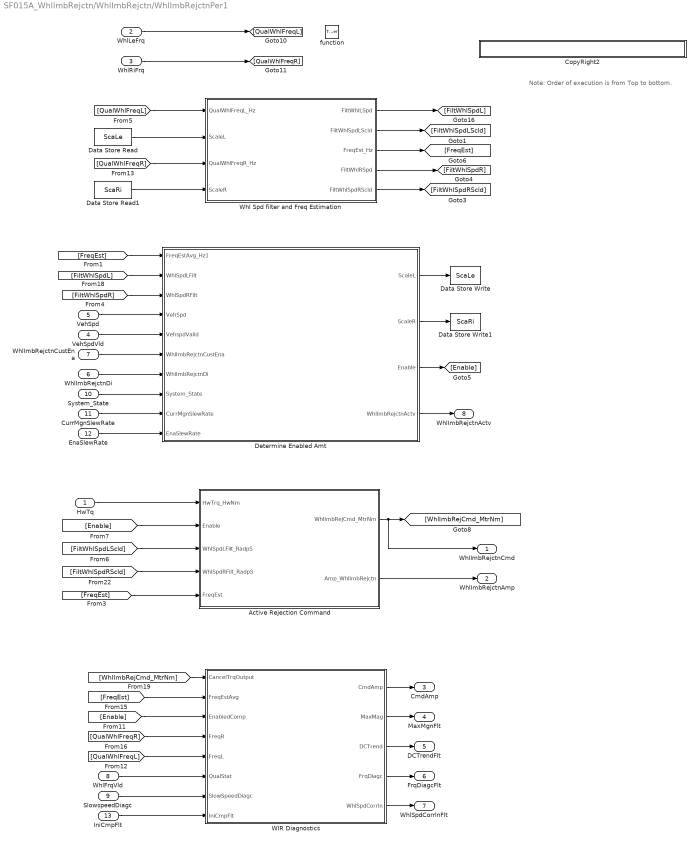
== system SF015A_WhlImbRejctn/WhlImbRejctn/WhlImbRejctnPer1 ==
  note: Note: Order of execution is from Top to bottom.
  HwTq : Inport
  WhlLeFrq : Inport  Port=2
  WhlRiFrq : Inport  Port=3
  VehSpdVld : Inport  Port=4
  VehSpd : Inport  Port=5
  WhlImbRejctnDi : Inport  Port=6
  WhlImbRejctnCustEna : Inport  Port=7
  WhlFrqVld : Inport  Port=8
  SlowspeedDiagc : Inport  Port=9
  System_State : Inport  Port=10
  CurrMgnSlewRate : Inport  Port=11
  EnaSlewRate : Inport  Port=12
  IniCmpFlt : Inport  Port=13
  function : TriggerPort  TriggerType=function-call
  "Active Rejection Command " : Subsystem
  CopyRight2 : Subsystem  Description=|  mask(Copyright Information){none=on}
      | Copyright info block.                                               
      |                                                                     
      | Place copyright information at the top of every subsystem in design.
      mask prompts: none "No parameters"
      mask help: Place copyright information at the top of every subsystem in design.
      mask Display:
      | NxtrConf = 'Nexteer Confidential';
      | 
      | sys = bdroot; %handle for the current model ("system")
      | first = get_param(sys,'Created');
      | first = first(end-3:end);  %year is last four digits
      | 
      | last = get_param(sys,'LastModifiedDate');
      | if isempty(last)
      |     last = datestr(now,'yyyy');
      | else
      |     last = last(end-3:end);
      | end
      | 
      | if strcmp(first,last)
      |     fprintf('%s -- Copyright %s Nexteer',NxtrConf,first)
      | else
      |     fprintf('%s -- %s%s- %s Nexteer',NxtrConf,char(169),first,last)
      | end
  Data Store Read : DataStoreRead  Priority=1  DataStoreName=ScaLe
      settings: AttributesFormatString=%<Priority>
  Data Store Read1 : DataStoreRead  Priority=1  DataStoreName=ScaRi
      settings: AttributesFormatString=%<Priority>
  Data Store Write : DataStoreWrite  Priority=2  DataStoreName=ScaLe
      settings: AttributesFormatString=%<Priority>
  Data Store Write1 : DataStoreWrite  Priority=2  DataStoreName=ScaRi
      settings: AttributesFormatString=%<Priority>
  Determine Enabled Amt : Subsystem
  WIR Diagnostics : Subsystem
  Whl Spd filter and Freq Estimation : Subsystem
  WhlImbRejctnCmd : Outport
  WhlImbRejctnAmp : Outport  Port=2
  CmdAmp : Outport  Port=3
  MaxMgnFlt : Outport  Port=4
  DCTrendFlt : Outport  Port=5
  FrqDiagcFlt : Outport  Port=6
  WhlSpdCorrlnFlt : Outport  Port=7
  WhlImbRejctnActv : Outport  Port=8
  wires:
  Determine Enabled Amt/3(Enable) -> [Enable]
  WhlLeFrq/1 -> [QualWhlFreqL]
  [FiltWhlSpdRScld] -> "Active Rejection Command "/4(WhlSpdRFilt_RadpS)
  "Active Rejection Command "/1(WhlImbRejCmd_MtrNm) -> WhlImbRejctnCmd/1, [WhlImbRejCmd_MtrNm]
  Determine Enabled Amt/2(ScaleR) -> Data Store Write1/1
  Whl Spd filter and Freq Estimation/1(FiltWhlLSpd) -> [FiltWhlSpdL]
  Whl Spd filter and Freq Estimation/4(FiltWhlRSpd) -> [FiltWhlSpdR]
  Data Store Read1/1 -> Whl Spd filter and Freq Estimation/4(ScaleR)
  HwTq/1 -> "Active Rejection Command "/1(HwTrq_HwNm)
  Whl Spd filter and Freq Estimation/5(FiltWhlSpdRScld) -> [FiltWhlSpdRScld]
  Data Store Read/1 -> Whl Spd filter and Freq Estimation/2(ScaleL)
  [FiltWhlSpdR] -> Determine Enabled Amt/3(WhlSpdRFilt)
  Determine Enabled Amt/1(ScaleL) -> Data Store Write/1
  VehSpd/1 -> Determine Enabled Amt/4(VehSpd)
  [FiltWhlSpdL] -> Determine Enabled Amt/2(WhlSpdLFilt)
  [FiltWhlSpdLScld] -> "Active Rejection Command "/3(WhlSpdLFilt_RadpS)
  [Enable] -> "Active Rejection Command "/2(Enable)
  Whl Spd filter and Freq Estimation/2(FiltWhlSpdLScld) -> [FiltWhlSpdLScld]
  "Active Rejection Command "/2(Amp_WhlImbRejctn) -> WhlImbRejctnAmp/1
  WhlRiFrq/1 -> [QualWhlFreqR]
  VehSpdVld/1 -> Determine Enabled Amt/5(VehspdValid)
  WhlImbRejctnCustEna/1 -> Determine Enabled Amt/6(WhlImbRejctnCustEna)
  WhlImbRejctnDi/1 -> Determine Enabled Amt/7(WhlImbRejctnDi)
  Whl Spd filter and Freq Estimation/3(FreqEst_Hz) -> [FreqEst]
  [FreqEst] -> Determine Enabled Amt/1(FreqEstAvg_Hz1)
  [FreqEst] -> "Active Rejection Command "/5(FreqEst)
  [WhlImbRejCmd_MtrNm] -> WIR Diagnostics/1(CancelTrqOutput)
  [FreqEst] -> WIR Diagnostics/2(FreqEstAvg)
  [Enable] -> WIR Diagnostics/3(EnabledComp)
  [QualWhlFreqR] -> WIR Diagnostics/4(FreqR)
  [QualWhlFreqL] -> WIR Diagnostics/5(FreqL)
  WhlFrqVld/1 -> WIR Diagnostics/6(QualStat)
  WIR Diagnostics/1(CmdAmp) -> CmdAmp/1
  SlowspeedDiagc/1 -> WIR Diagnostics/7("SlowSpeedDiagc ")
  System_State/1 -> Determine Enabled Amt/8(System_State)
  WIR Diagnostics/2(MaxMag) -> MaxMgnFlt/1
  WIR Diagnostics/3(DCTrend) -> DCTrendFlt/1
  WIR Diagnostics/4(FrqDiagc) -> FrqDiagcFlt/1
  WIR Diagnostics/5(WhlSpdCorrln) -> WhlSpdCorrlnFlt/1
  [QualWhlFreqL] -> Whl Spd filter and Freq Estimation/1(QualWhlFreqL_Hz)
  [QualWhlFreqR] -> Whl Spd filter and Freq Estimation/3(QualWhlFreqR_Hz)
  Determine Enabled Amt/4(WhlImbRejctnActv) -> WhlImbRejctnActv/1
  CurrMgnSlewRate/1 -> Determine Enabled Amt/9(CurrMgnSlewRate)
  EnaSlewRate/1 -> Determine Enabled Amt/10(EnaSlewRate)
  IniCmpFlt/1 -> WIR Diagnostics/8(IniCmpFlt)

== system SF015A_WhlImbRejctn/WhlImbRejctn/WhlImbRejctnPer2 ==
  CmdAmp : Inport
  MaxMag : Inport  Port=2
  DcTrend : Inport  Port=3
  FrqDiagc : Inport  Port=4
  WhlSpdCorrln : Inport  Port=5
  function : TriggerPort  TriggerType=function-call
  Constant12 : Constant  Value=WhlImbRejctnWhlSpdCorrlnFltRcvryDly
  Constant5 : Constant  Value=WhlImbRejctnMaxMgnFltRcvryDly
  Constant6 : Constant  Value=WhlImbRejctnDcTrendFltRcvryDly
  Constant9 : Constant  Value=WhlImbRejctnFrqDiagcFltRcvryDly
  CopyRight2 : Subsystem  Description=|  mask(Copyright Information){none=on}
      | Copyright info block.                                               
      |                                                                     
      | Place copyright information at the top of every subsystem in design.
      mask prompts: none "No parameters"
      mask help: Place copyright information at the top of every subsystem in design.
      mask Display:
      | NxtrConf = 'Nexteer Confidential';
      | 
      | sys = bdroot; %handle for the current model ("system")
      | first = get_param(sys,'Created');
      | first = first(end-3:end);  %year is last four digits
      | 
      | last = get_param(sys,'LastModifiedDate');
      | if isempty(last)
      |     last = datestr(now,'yyyy');
      | else
      |     last = last(end-3:end);
      | end
      | 
      | if strcmp(first,last)
      |     fprintf('%s -- Copyright %s Nexteer',NxtrConf,first)
      | else
      |     fprintf('%s -- %s%s- %s Nexteer',NxtrConf,char(169),first,last)
      | end
  Flt Recovery- DC Trend : Subsystem
  Flt Recovery- Freq Diag : Subsystem
  Flt Recovery- Max Mag : Subsystem
  Flt Recovery- WhlSpdCorr Diag : Subsystem
  WIR Low Speed Diagnostics : Subsystem
  "SlowSpeedDiagc " : Outport
  wires:
  Constant5/1 -> Flt Recovery- Max Mag/2(FltRecDly)
  MaxMag/1 -> Flt Recovery- Max Mag/1(FltStatIn)
  Constant6/1 -> Flt Recovery- DC Trend/2(FltRecDly)
  Constant9/1 -> Flt Recovery- Freq Diag/2(FltRecDly)
  Constant12/1 -> Flt Recovery- WhlSpdCorr Diag/2(FltRecDly)
  DcTrend/1 -> Flt Recovery- DC Trend/1(FltStatIn)
  FrqDiagc/1 -> Flt Recovery- Freq Diag/1(FltStatIn)
  WhlSpdCorrln/1 -> Flt Recovery- WhlSpdCorr Diag/1(FltStatIn)
  CmdAmp/1 -> WIR Low Speed Diagnostics/1(CmdAmp)
  WIR Low Speed Diagnostics/1(WIRFltStatus_SlowSpeed) -> "SlowSpeedDiagc "/1
